simulink model "task2_7"  (R2015b)
settings: Solver=ode45  StartTime=tstart  StopTime=tstop  RelTol=1e-3
values from neighbouring files (symbols this model uses):
  c = 0    [run_27_.m]    (also in run_2_7.m = 1)
  D2T = 500    [run_2_7.m]
  DELTA_p = 1300    [run_2_7.m]
  I_max = 0.06    [run_2_7.m]
  Ki_LOS = 2e-6    (= 2e-06)    [run_2_7.m]
  psi0 = 0    [run_27_.m]    (also in run_2_7.m)
  R = [cos(psiTemp) -sin(psiTemp); sin(psiTemp) cos(psiTemp)]    [pathplotter.m]    (also in run_27_.m = 1200; run_2_7.m = 1200)
  r0 = 0    [run_27_.m]    (also in run_2_7.m)
  tsamp = 10    [run_27_.m]    (also in run_2_7.m)
  U_a_max = 4    [run_2_7.m]
  v0 = [6.63 0]'    [run_27_.m]    (also in run_2_7.m)
  V_t = [3*cos(psi_T) ; 3*sin(psi_T)]    [run_2_7.m]
  w_u = 0.06    [run_2_7.m]
undefined symbols (not defined in the file or in its folder): delta_max, k_b0, kd_psi, ki_psi, Ki_u, kp_psi, Kp_u, msfartoystyring, n_c_k, n_c_max, n_dot_max, w_psi, WP
undefined symbols (not defined in the file): p0
settings Model: ExtModeAutoUpdateStatusClock=off  Creator=christh  LastModifiedBy=Erik
settings DataIOCC: SaveFormat=Array  SignalLoggingSaveFormat=ModelDataLogs
settings OptimizationCC: ExpressionDepthLimit=2147483647  InitFltsAndDblsToZero=on
settings DebuggingCC: UnderspecifiedInitializationDetection=Classic  MergeDetectMultiDrivingBlocksExec=none  SolverPrmCheckMsg=warning  FcnCallInpInsideContextMsg=UseLocalSettings  StateNameClashWarn=warning
settings HardwareCC: ProdBitPerPointer=32  ProdLargestAtomicFloat=None  ProdIntDivRoundTo=Undefined  ProdEndianess=Unspecified  ProdWordSize=32  ProdHWDeviceType=32-bit Generic
settings GRTTargetCC: GeneratePreprocessorConditionals=Disable all  CombineOutputUpdateFcns=off  GRTInterface=on
settings ConfigComp: CovModelRefEnable=Off

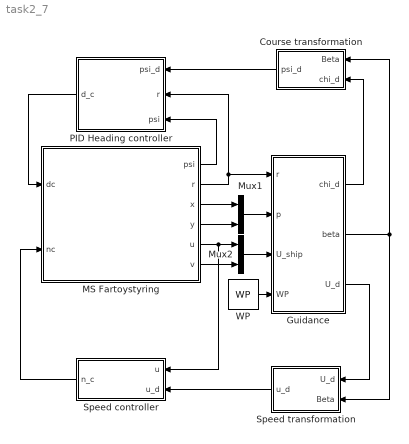
== system task2_7 ==
  Course transformation : Subsystem
  Guidance : Subsystem
  MS Fartoystyring : Subsystem  mask(MS Fartoystyring for Assignment 3 G&C){x0=p0(1), y0=p0(2), u0=v0(1), v0=v0(2), psi0=psi0, r0=r0, c=c}
      mask prompts: x0 "x(t0) (m)"; y0 "y(t0) (m)"; u0 "u(t0) (m/s)"; v0 "v(t0) (m/s)"; psi0 "psi(t0) (rad)"; r0 "r(t0) (rad/s)"; c "current (0 or 1)"
      mask help:
      | Block corresponding to Figure 1 in the assignment text. Gives the response of the ship.
      |
      | The design speed of MS Fartoystyring is u=8.23 m/s.
      |
      | Input:
      | dc: commanded rudder (rad), dmax=25*pi/180
      | nc: commanded shaft speed (rad/s), nmax=85*2*pi/60
      |
      | Output:
      | x: north pos (m)
      | y: east pos (m)
      | u: surge (m/s)
      | v: sway (m/s)
      | psi: heading (rad)
      | r: yaw (rad/s)
      mask Help: Comments, bugs and help requests can be directed to the TA. Email on course website.
  Mux1 : Mux  Inputs=2
  Mux2 : Mux  Inputs=2
  PID Heading controller : Subsystem
  Speed controller : Subsystem
  Speed transformation : Subsystem
  WP : Constant  Value=WP
  wires:
  MS Fartoystyring/1(psi) -> PID Heading controller/3(psi)
  MS Fartoystyring/2(r) -> Guidance/1(r), PID Heading controller/2(r)
  MS Fartoystyring/3(x) -> Mux1/1
  MS Fartoystyring/4(y) -> Mux1/2
  Mux1/1 -> Guidance/2(p)
  MS Fartoystyring/5(u) -> Speed controller/1(u), Mux2/1
  PID Heading controller/1(d_c) -> MS Fartoystyring/1(dc)
  MS Fartoystyring/6(v) -> Mux2/2
  Mux2/1 -> Guidance/3(U_ship)
  WP/1 -> Guidance/4(WP)
  Guidance/1(chi_d) -> Course transformation/2(chi_d)
  Guidance/3(U_d) -> Speed transformation/1(U_d)
  Guidance/2(beta) -> Speed transformation/2(Beta), Course transformation/1(Beta)
  Speed transformation/1(u_d) -> Speed controller/2(u_d)
  Course transformation/1(psi_d) -> PID Heading controller/1(psi_d)
  Speed controller/1(n_c) -> MS Fartoystyring/2(nc)

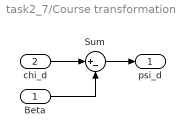
== system task2_7/Course transformation ==
  Beta : Inport
  chi_d : Inport  Port=2
  Sum : Sum  Inputs=|+-
  psi_d : Outport
  wires:
  chi_d/1 -> Sum/1
  Beta/1 -> Sum/2
  Sum/1 -> psi_d/1

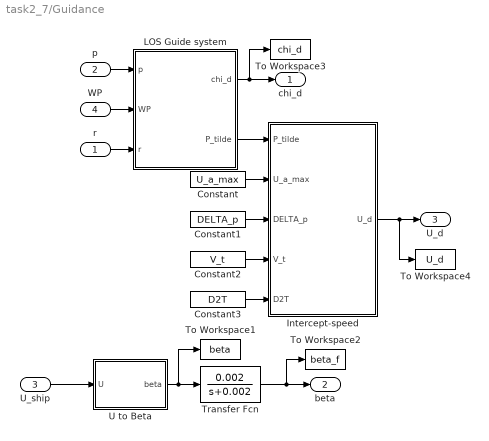
== system task2_7/Guidance ==
  r : Inport
  p : Inport  Port=2
  U_ship : Inport  Port=3
  WP : Inport  Port=4
  Constant : Constant  Value=U_a_max
  Constant1 : Constant  Value=DELTA_p
  Constant2 : Constant  Value=V_t
  Constant3 : Constant  Value=D2T
  Intercept-speed : MATLAB Function  TreatAsAtomicUnit=on
  LOS Guide system : Subsystem  Description=LOS
  To Workspace1 : ToWorkspace  VariableName=beta  SampleTime=tsamp
  To Workspace2 : ToWorkspace  VariableName=beta_f  SampleTime=tsamp
  To Workspace3 : ToWorkspace  VariableName=chi_d  SampleTime=tsamp
  To Workspace4 : ToWorkspace  VariableName=U_d  SampleTime=tsamp
  Transfer Fcn : TransferFcn  Numerator=[0.002]  Denominator=[1 0.002]
  U to Beta : MATLAB Function  TreatAsAtomicUnit=on
  chi_d : Outport
  beta : Outport  Port=2
  U_d : Outport  Port=3
  wires:
  U_ship/1 -> U to Beta/1(U)
  p/1 -> LOS Guide system/1(p)
  WP/1 -> LOS Guide system/2(WP)
  Constant/1 -> Intercept-speed/2(U_a_max)
  Constant1/1 -> Intercept-speed/3(DELTA_p)
  U to Beta/1(beta) -> Transfer Fcn/1, To Workspace1/1
  LOS Guide system/2(P_tilde) -> Intercept-speed/1(P_tilde)
  LOS Guide system/1(chi_d) -> To Workspace3/1, chi_d/1
  Constant2/1 -> Intercept-speed/4(V_t)
  Intercept-speed/1(U_d) -> To Workspace4/1, U_d/1
  Transfer Fcn/1 -> To Workspace2/1, beta/1
  Constant3/1 -> Intercept-speed/5(D2T)
  r/1 -> LOS Guide system/3(r)

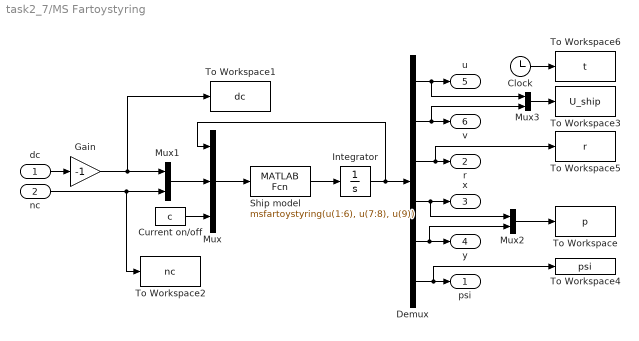
== system task2_7/MS Fartoystyring ==
  dc : Inport
  nc : Inport  Port=2
  Clock : Clock
  Current on/off : Constant  Value=c
  Demux : Demux  Outputs=6
  Gain : Gain  Gain=-1
  Integrator : Integrator  InitialCondition=[u0 v0 r0 x0 y0 psi0]'
  Mux : Mux  Inputs=3
  Mux1 : Mux  Inputs=2
  Mux2 : Mux  Inputs=2
  Mux3 : Mux  Inputs=2
  Ship model : MATLABFcn  MATLABFcn=msfartoystyring(u(1:6), u(7:8), u(9))  OutputDimensions=6
  To Workspace : ToWorkspace  VariableName=p  SampleTime=tsamp
  To Workspace1 : ToWorkspace  VariableName=dc  SampleTime=tsamp
  To Workspace2 : ToWorkspace  VariableName=nc  SampleTime=tsamp
  To Workspace3 : ToWorkspace  VariableName=U_ship  SampleTime=tsamp
  To Workspace4 : ToWorkspace  VariableName=psi  SampleTime=tsamp
  To Workspace5 : ToWorkspace  VariableName=r  SampleTime=tsamp
  To Workspace6 : ToWorkspace  VariableName=t  SampleTime=tsamp
  psi : Outport
  r : Outport  Port=2
  x : Outport  Port=3
  y : Outport  Port=4
  u : Outport  Port=5
  v : Outport  Port=6
  wires:
  Integrator/1 -> Mux/1, Demux/1
  Mux1/1 -> Mux/2
  dc/1 -> Gain/1
  nc/1 -> Mux1/2, To Workspace2/1
  Demux/1 -> Mux3/1, u/1
  Demux/2 -> Mux3/2, v/1
  Demux/3 -> To Workspace5/1, r/1
  Demux/4 -> Mux2/1, x/1
  Demux/5 -> y/1, Mux2/2
  Demux/6 -> To Workspace4/1, psi/1
  Current on/off/1 -> Mux/3
  Ship model/1 -> Integrator/1
  Mux/1 -> Ship model/1
  Mux2/1 -> To Workspace/1
  Clock/1 -> To Workspace6/1
  Mux3/1 -> To Workspace3/1
  Gain/1 -> To Workspace1/1, Mux1/1

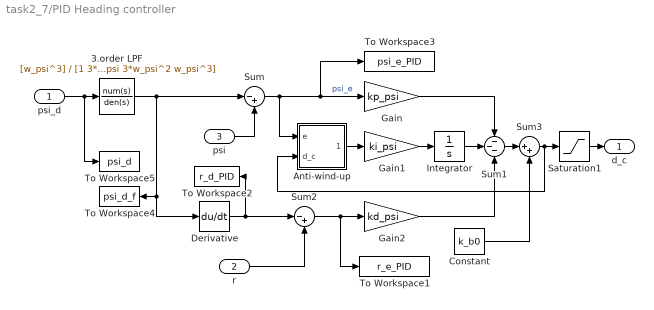
== system task2_7/PID Heading controller ==
  psi_d : Inport
  r : Inport  Port=2
  psi : Inport  Port=3
  3.order LPF : TransferFcn  Numerator=[w_psi^3]  Denominator=[1 3*w_psi 3*w_psi^2 w_psi^3]
  Anti-wind-up : MATLAB Function  TreatAsAtomicUnit=on
  Constant : Constant  Value=k_b0
  Derivative : Derivative
  Gain : Gain  Gain=kp_psi
  Gain1 : Gain  Gain=ki_psi
  Gain2 : Gain  Gain=kd_psi
  Integrator : Integrator
  Saturation1 : Saturate  UpperLimit=delta_max  LowerLimit=-delta_max
  Sum : Sum  Inputs=|-+
  Sum1 : Sum  Inputs=---
  Sum2 : Sum  Inputs=|-+
  Sum3 : Sum  Inputs=|++
  To Workspace1 : ToWorkspace  VariableName=r_e_PID  SampleTime=tsamp
  To Workspace2 : ToWorkspace  VariableName=r_d_PID  SampleTime=tsamp
  To Workspace3 : ToWorkspace  VariableName=psi_e_PID  SampleTime=tsamp
  To Workspace4 : ToWorkspace  VariableName=psi_d_f  SampleTime=tsamp
  To Workspace5 : ToWorkspace  VariableName=psi_d  SampleTime=tsamp
  d_c : Outport
  wires:
  Saturation1/1 -> d_c/1
  Sum3/1 -> Anti-wind-up/2(d_c), Saturation1/1
  psi/1 -> Sum/2
  Sum/1 -> Anti-wind-up/1(e), Gain/1, To Workspace3/1  "psi_e"
  Gain1/1 -> Integrator/1
  Gain/1 -> Sum1/1
  Integrator/1 -> Sum1/2
  Gain2/1 -> Sum1/3
  Sum1/1 -> Sum3/1
  Constant/1 -> Sum3/2
  Sum2/1 -> To Workspace1/1, Gain2/1
  r/1 -> Sum2/2
  Derivative/1 -> Sum2/1, To Workspace2/1
  psi_d/1 -> To Workspace5/1, 3.order LPF/1
  3.order LPF/1 -> Derivative/1, To Workspace4/1, Sum/1
  Anti-wind-up/1(e_out) -> Gain1/1

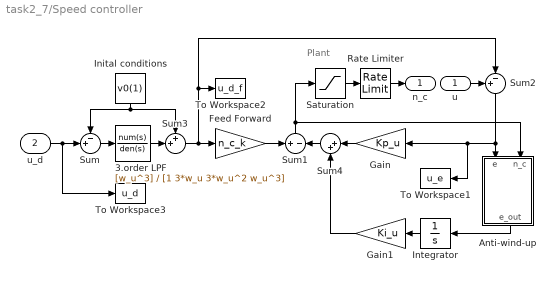
== system task2_7/Speed controller ==
  note: Plant
  u : Inport
  u_d : Inport  Port=2
  3.order LPF : TransferFcn  Numerator=[w_u^3]  Denominator=[1 3*w_u 3*w_u^2 w_u^3]
  Anti-wind-up : MATLAB Function  TreatAsAtomicUnit=on
  Feed Forward : Gain  Gain=n_c_k
  Gain : Gain  Gain=Kp_u
  Gain1 : Gain  Gain=Ki_u
  Inital conditions : Constant  Value=v0(1)
  Integrator : Integrator
  Rate Limiter : RateLimiter  RisingSlewLimit=n_dot_max  FallingSlewLimit=-n_dot_max
  Saturation : Saturate  UpperLimit=n_c_max  LowerLimit=0.2
  Sum : Sum  Inputs=-+|
  Sum1 : Sum  Inputs=+-
  Sum2 : Sum  Inputs=+-|
  Sum3 : Sum  Inputs=++|
  Sum4 : Sum  Inputs=|++
  To Workspace1 : ToWorkspace  VariableName=u_e  SampleTime=tsamp
  To Workspace2 : ToWorkspace  VariableName=u_d_f  SampleTime=tsamp
  To Workspace3 : ToWorkspace  VariableName=u_d  SampleTime=tsamp
  n_c : Outport
  wires:
  Sum1/1 -> Anti-wind-up/2(n_c), Saturation/1
  Saturation/1 -> Rate Limiter/1
  Rate Limiter/1 -> n_c/1
  u_d/1 -> Sum/2, To Workspace3/1
  Feed Forward/1 -> Sum1/1
  u/1 -> Sum2/1
  Sum2/1 -> To Workspace1/1, Gain/1, Anti-wind-up/1(e)
  Sum/1 -> 3.order LPF/1
  Inital conditions/1 -> Sum/1, Sum3/1
  3.order LPF/1 -> Sum3/2
  Sum3/1 -> Sum2/2, To Workspace2/1, Feed Forward/1
  Integrator/1 -> Gain1/1
  Sum4/1 -> Sum1/2
  Gain/1 -> Sum4/1
  Gain1/1 -> Sum4/2
  Anti-wind-up/1(e_out) -> Integrator/1

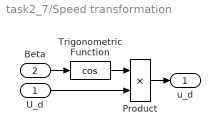
== system task2_7/Speed transformation ==
  U_d : Inport
  Beta : Inport  Port=2
  Product : Product
  Trigonometric Function : Trigonometry  Operator=cos
  u_d : Outport
  wires:
  Product/1 -> u_d/1
  Beta/1 -> Trigonometric Function/1
  U_d/1 -> Product/2
  Trigonometric Function/1 -> Product/1

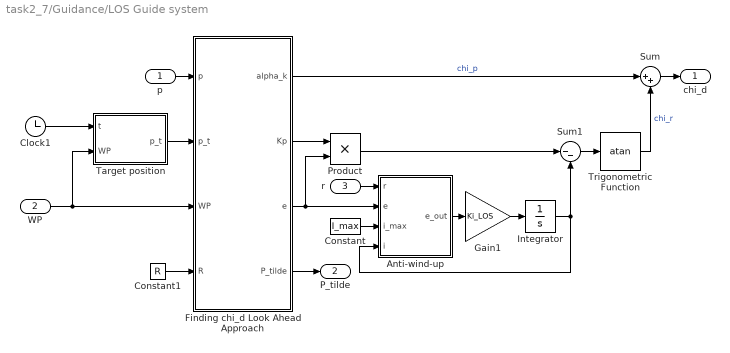
== system task2_7/Guidance/LOS Guide system ==
  p : Inport
  WP : Inport  Port=2
  r : Inport  Port=3
  Anti-wind-up : MATLAB Function  TreatAsAtomicUnit=on
  Clock1 : Clock
  Constant : Constant  Value=I_max
  Constant1 : Constant  Value=R
  Finding chi_d Look Ahead Approach : MATLAB Function  TreatAsAtomicUnit=on
  Gain1 : Gain  Gain=Ki_LOS
  Integrator : Integrator
  Product : Product
  Sum : Sum  Inputs=|++
  Sum1 : Sum  Inputs=|--
  Target position : MATLAB Function  TreatAsAtomicUnit=on
  Trigonometric Function : Trigonometry  Operator=atan
  chi_d : Outport
  P_tilde : Outport  Port=2
  wires:
  WP/1 -> Target position/2(WP), Finding chi_d Look Ahead Approach/3(WP)
  p/1 -> Finding chi_d Look Ahead Approach/1(p)
  Constant1/1 -> Finding chi_d Look Ahead Approach/4(R)
  Sum1/1 -> Trigonometric Function/1
  Finding chi_d Look Ahead Approach/3(e) -> Anti-wind-up/2(e), Product/2
  Finding chi_d Look Ahead Approach/1(alpha_k) -> Sum/1  "chi_p"
  Product/1 -> Sum1/1
  Trigonometric Function/1 -> Sum/2  "chi_r"
  Sum/1 -> chi_d/1
  Integrator/1 -> Anti-wind-up/4(i), Sum1/2
  Constant/1 -> Anti-wind-up/3(i_max)
  Finding chi_d Look Ahead Approach/2(Kp) -> Product/1
  Target position/1(p_t) -> Finding chi_d Look Ahead Approach/2(p_t)
  Clock1/1 -> Target position/1(t)
  Finding chi_d Look Ahead Approach/4(P_tilde) -> P_tilde/1
  r/1 -> Anti-wind-up/1(r)
  Anti-wind-up/1(e_out) -> Gain1/1
  Gain1/1 -> Integrator/1

== matlab function task2_7/Guidance/Intercept-speed ==
  data: P_tilde input; U_a_max input; DELTA_p input; V_t input; U_d output; D2T input
function U_d = fcn(P_tilde,U_a_max, DELTA_p,V_t, D2T)
kapa = U_a_max * (norm(P_tilde) - D2T)/sqrt(P_tilde'*P_tilde + DELTA_p^2);
V_a = -kapa * P_tilde/norm(P_tilde);
V_d = V_t + V_a;
U_d = norm(V_d);
end

== matlab function task2_7/Guidance/LOS Guide system/Finding chi_d Look Ahead Approach ==
  data: p input; p_t input; alpha_k output; WP input; Kp output; e output; P_tilde output; R input
function [alpha_k, Kp, e, P_tilde] = fcn(p,p_t, WP, R)

    persistent index;

    if isempty(index)
         index = 2;
    end

    % The craft's position in NED
    x = p(1);   %[m] 
    y = p(2);   %[m]    

    % The next and previous waypoint in NED
    xk = WP(1, index - 1);                  xk_1 = WP(1, index); 
    yk = WP(2, index - 1);                  yk_1 = WP(2, index);

    % How far from the desired waypoint the craft must be before going to next waypoint
    % turning_Radius = 500; 
    % 
    % if (((xk_1 - x)^2 + (yk_1 - y)^2) <= turning_Radius^2) && (length(WP) > index)  
    %     index = index + 1;
    % end

    %The angle between the North and two waypoints --> atan2(dy/dx)
    alpha_k =  atan2(yk_1 - yk, xk_1 - xk); %[rad] 

    %The rotation from the NED frame to path-fixed reference frame
    Rp = [  cos(alpha_k)   -sin(alpha_k);
            sin(alpha_k)   cos(alpha_k);];

    %How far the craft is from the previous way point
    p_tilde = [x,y]' - [xk,yk]'; % or p-WP_previous
    
    %Position vector to intercepting vessen
   P_tilde = p-p_t;

    % The coordinates of the craft in the path-fixed reference frame (Fossen
    % p258)
    Epsilon = Rp' * p_tilde;

    % Along track distance & cross track error
    s = Epsilon(1,:);
    e = Epsilon(2,:);

    %The look ahead distance DELTA
    if R > abs(e)
        DELTA = sqrt((R^2-e^2));
    else
        DELTA = NaN;
    end

    % Steering law
    if (~isnan(DELTA)) && (DELTA ~=0)
        Kp = 1/DELTA;
    else
        Kp = 0.013;
    end
end

== matlab function task2_7/Guidance/U to Beta ==
  data: U input; beta output
function beta = fcn(U)
u = U(1);
v = U(2);
beta = asin(v/sqrt(u^2 +v^2));
end

== matlab function task2_7/Speed controller/Anti-wind-up ==
  data: e input; e_out output; n_c input
function e_out = fcn(e, n_c)
    n_c_max = 8.9; 
    if n_c >= n_c_max
        e_out = 0;
    else
        e_out = e;
    end
end

== matlab function task2_7/Guidance/LOS Guide system/Target position ==
  data: t input; p_t output; WP input
function p_t = fcn(t, WP)
psiTemp=atan2(WP(2,2)-WP(2,1),WP(1,2)-WP(1,1));
p_t = [ WP(1,2)+3*cos(psiTemp)*t ; WP(2,2)+3*sin(psiTemp)*t ];
end

== matlab function task2_7/Guidance/LOS Guide system/Anti-wind-up ==
  data: r input; e input; i_max input; e_out output; i input
function e_out = fcn(r,e,i_max, i)
if (abs(r) > 0.003) || (abs(e) > 200)
    e_out = 0;
elseif (i > i_max && e>0) || (i < -i_max && e<0)
    e_out = e/(5+4*abs(i)/i_max);
else
    e_out = e;
end
end

== matlab function task2_7/PID Heading controller/Anti-wind-up ==
  data: e input; e_out output; d_c input
function e_out = fcn(e, d_c)
    d_c_max = 0.4363;
    if d_c >= d_c_max
        e_out = 0;
    else
        e_out = e;
    end
end
